simulink model "Team_4_Project_1_sim_Saumil"  (R2021b)
settings: Solver=VariableStepAuto  StartTime=0.0  StopTime=1  RelTol=1e-3
undefined symbols (not defined in the file): D, K, l, mass, r, Small_k, x0
settings Model: Creator=saumilpradhan  LastModifiedBy=saumilpradhan

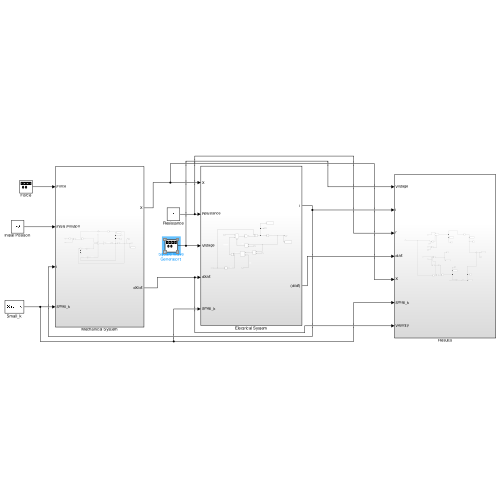
[thumbnail: Simulink's stored preview of the top-level diagram]
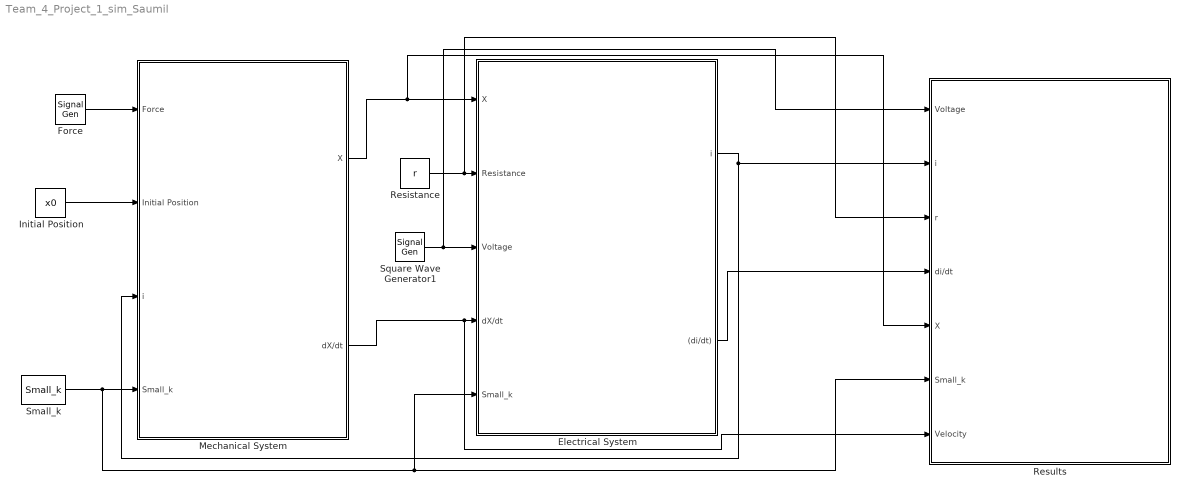
== system Team_4_Project_1_sim_Saumil ==
  Electrical System : Subsystem
  Force : SignalGenerator  WaveForm=square  Amplitude=4  Units=rad/sec
  Initial Position : Constant  Value=x0
  Mechanical System : Subsystem
  Resistance : Constant  Value=r
  Results : Subsystem
  Small_k : Constant  Value=Small_k
  Square Wave Generator1 : SignalGenerator  WaveForm=square  Amplitude=5
  wires:
  Mechanical System/2(dX/dt) -> Results/7(Velocity), Electrical System/4(dX/dt)
  Electrical System/1(i) -> Mechanical System/3(i), Results/2(i)
  Small_k/1 -> Results/6(Small_k), Electrical System/5(Small_k), Mechanical System/4(Small_k)
  Resistance/1 -> Results/3(r), Electrical System/2(Resistance)
  Mechanical System/1(X) -> Electrical System/1(X), Results/5(X)
  Initial Position/1 -> Mechanical System/2(Initial Position)
  Force/1 -> Mechanical System/1(Force)
  Square Wave Generator1/1 -> Results/1(Voltage), Electrical System/3(Voltage)
  Electrical System/2((di/dt)) -> Results/4(di/dt)

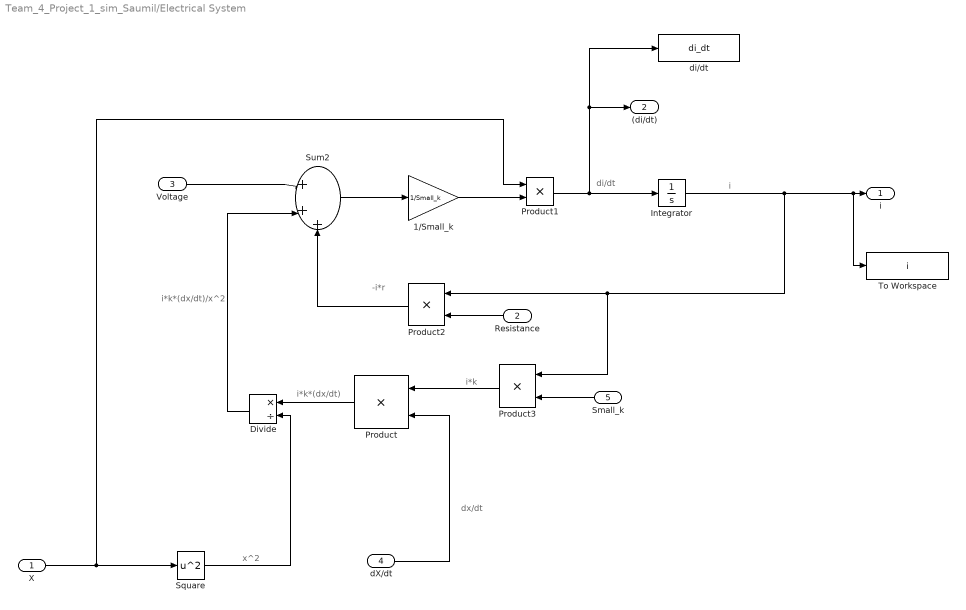
== system Team_4_Project_1_sim_Saumil/Electrical System ==
  note: dx/dt
  note: x^2
  note: i
  note: i*k
  note: i*k*(dx/dt)
  note: i*k*(dx/dt)/x^2
  note: -i*r
  note: di/dt
  X : Inport
  Resistance : Inport  Port=2
  Voltage : Inport  Port=3
  dX/dt : Inport  Port=4
  Small_k : Inport  Port=5
  1/Small_k : Gain  Gain=1/Small_k
  Divide : Product  Inputs=*/
  Integrator : Integrator
  Product{,1..3} (4 alike) : Product
  Square : Math  Operator=square  SaturateOnIntegerOverflow=on
  Sum2 : Sum  Inputs=|+++
  To Workspace : ToWorkspace  VariableName=i  SampleTime=-1
  di/dt : ToWorkspace  VariableName=di_dt  SampleTime=-1
  i : Outport
  (di/dt) : Outport  Port=2
  wires:
  Product3/1 -> Product/1
  Sum2/1 -> 1/Small_k/1
  dX/dt/1 -> Product/2
  Product/1 -> Divide/1
  Integrator/1 -> To Workspace/1, i/1, Product3/1, Product2/1
  Voltage/1 -> Sum2/1
  Divide/1 -> Sum2/2
  X/1 -> Product1/1, Square/1
  Square/1 -> Divide/2
  Product1/1 -> di/dt/1, (di/dt)/1, Integrator/1
  1/Small_k/1 -> Product1/2
  Product2/1 -> Sum2/3
  Resistance/1 -> Product2/2
  Small_k/1 -> Product3/2

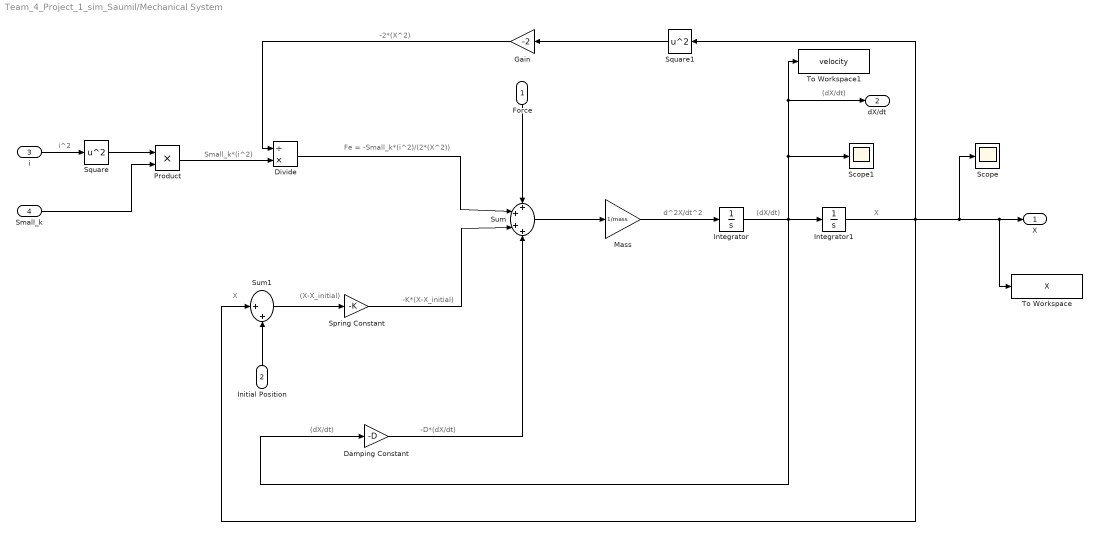
== system Team_4_Project_1_sim_Saumil/Mechanical System ==
  note: -D*(dX/dt)
  note: (X-X_initial)
  note: (dX/dt)
  note: -K*(X-X_initial)
  note: d^2X/dt^2
  note: (dX/dt)
  note: X
  note: X
  note: (dX/dt)
  note: i^2
  note: -2*(X^2)
  note: Small_k*(i^2)
  note: Fe = -Small_k*(i^2)/(2*(X^2))
  Force : Inport
  Initial Position : Inport  Port=2
  i : Inport  Port=3
  Small_k : Inport  Port=4
  Damping Constant : Gain  Gain=-D
  Divide : Product  Inputs=/*
  Gain : Gain  Gain=-2
  Integrator : Integrator
  Integrator1 : Integrator  InitialCondition=0.000001
  Mass : Gain  Gain=1/mass
  Product : Product
  Scope : Scope
  Scope1 : Scope
  Spring Constant : Gain  Gain=-K
  Square : Math  Operator=square  SaturateOnIntegerOverflow=on
  Square1 : Math  Operator=square  SaturateOnIntegerOverflow=on
  Sum : Sum  Inputs=++++
  Sum1 : Sum  Inputs=|++
  To Workspace : ToWorkspace  VariableName=X  SampleTime=-1
  To Workspace1 : ToWorkspace  VariableName=velocity  SampleTime=-1
  X : Outport
  dX/dt : Outport  Port=2
  wires:
  Damping Constant/1 -> Sum/4
  Integrator/1 -> Scope1/1, To Workspace1/1, dX/dt/1, Damping Constant/1, Integrator1/1
  Initial Position/1 -> Sum1/2
  Force/1 -> Sum/1
  Integrator1/1 -> Sum1/1, Square1/1, Scope/1, To Workspace/1, X/1
  Sum1/1 -> Spring Constant/1
  Spring Constant/1 -> Sum/3
  Sum/1 -> Mass/1
  Mass/1 -> Integrator/1
  i/1 -> Square/1
  Square/1 -> Product/1
  Small_k/1 -> Product/2
  Product/1 -> Divide/2
  Square1/1 -> Gain/1
  Gain/1 -> Divide/1
  Divide/1 -> Sum/2

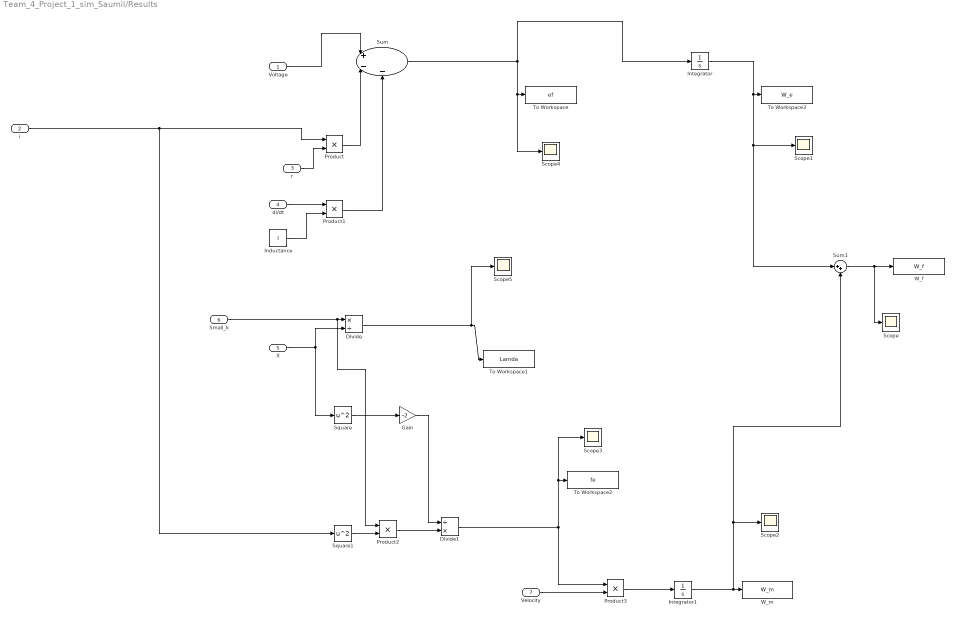
== system Team_4_Project_1_sim_Saumil/Results ==
  Voltage : Inport
  i : Inport  Port=2
  r : Inport  Port=3
  di/dt : Inport  Port=4
  X : Inport  Port=5
  Small_k : Inport  Port=6
  Velocity : Inport  Port=7
  Divide : Product  Inputs=*/
  Divide1 : Product  Inputs=/*
  Gain : Gain  Gain=-2
  Inductance : Constant  Value=l
  Integrator : Integrator
  Integrator1 : Integrator
  Product{,1..3} (4 alike) : Product
  Scope{,1..5} (6 alike) : Scope
  Square : Math  Operator=square  SaturateOnIntegerOverflow=on
  Square1 : Math  Operator=square  SaturateOnIntegerOverflow=on
  Sum : Sum  Inputs=|+--
  Sum1 : Sum  Inputs=|++
  To Workspace : ToWorkspace  VariableName=ef  SampleTime=-1
  To Workspace1 : ToWorkspace  VariableName=Lamda  SampleTime=-1
  To Workspace2 : ToWorkspace  VariableName=fe  SampleTime=-1
  To Workspace3 : ToWorkspace  VariableName=W_e  SampleTime=-1
  W_f : ToWorkspace  VariableName=W_f  SampleTime=-1
  W_m : ToWorkspace  VariableName=W_m  SampleTime=-1
  wires:
  i/1 -> Product/1, Square1/1
  r/1 -> Product/2
  Voltage/1 -> Sum/1
  Product/1 -> Sum/2
  di/dt/1 -> Product1/1
  Inductance/1 -> Product1/2
  Product1/1 -> Sum/3
  Sum/1 -> Scope4/1, To Workspace/1, Integrator/1
  Small_k/1 -> Product2/1, Divide/1
  Divide/1 -> Scope5/1, To Workspace1/1
  X/1 -> Square/1, Divide/2
  Divide1/1 -> Scope3/1, To Workspace2/1, Product3/1
  Square1/1 -> Product2/2
  Product2/1 -> Divide1/2
  Square/1 -> Gain/1
  Gain/1 -> Divide1/1
  Integrator/1 -> Sum1/1, Scope1/1, To Workspace3/1
  Velocity/1 -> Product3/2
  Product3/1 -> Integrator1/1
  Integrator1/1 -> Sum1/2, Scope2/1, W_m/1
  Sum1/1 -> Scope/1, W_f/1
